simulink model "Block Diagram"  (R2024b)
settings: Solver=VariableStepAuto  StartTime=0.0  StopTime=10.0  RelTol=1e-3
libraries: simulink_extras x43, eeGeneralControl x4
(part 1 of 3)
settings Model: Creator=uig55046  LastModifiedBy=deepo
settings RTWCC: GPUComputeCapability=3.5

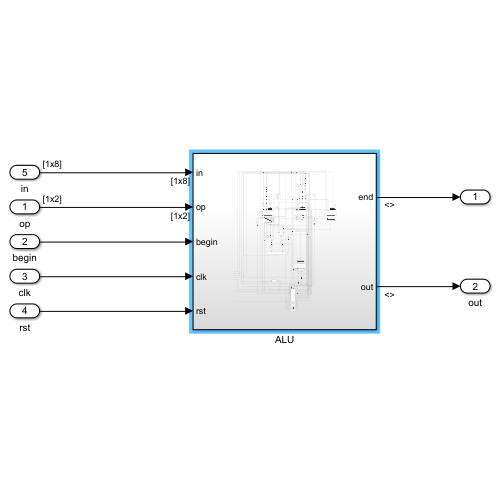
[thumbnail: Simulink's stored preview of the top-level diagram]
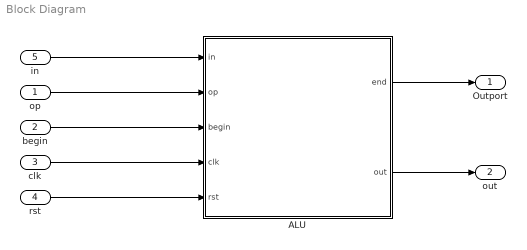
== system Block Diagram ==
  op : Inport  OutDataTypeStr=boolean  PortDimensions=[1 2]
  begin : Inport  Port=2  OutDataTypeStr=boolean  PortDimensions=[1]
      settings: VarSizeSig=Yes
  clk : Inport  Port=3  OutDataTypeStr=boolean  PortDimensions=1
  rst : Inport  Port=4
  in : Inport  Port=5  PortDimensions=[1 8]
  ALU : Subsystem
  Outport : Outport
  out : Outport  Port=2
  wires:
  op/1 -> ALU/2(op)
  begin/1 -> ALU/3(begin)
  clk/1 -> ALU/4(clk)
  ALU/1(end) -> Outport/1
  rst/1 -> ALU/5(rst)
  in/1 -> ALU/1(in)
  ALU/2(out) -> out/1

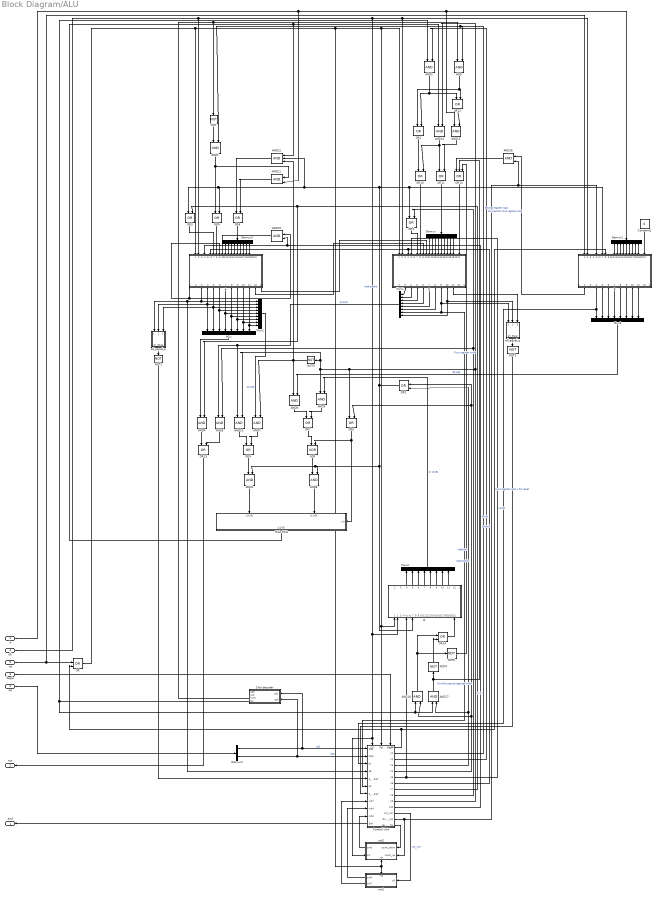
== system Block Diagram/ALU ==
  in : Inport  PortDimensions=[1 8]
  op : Inport  Port=2  PortDimensions=[1 2]
  begin : Inport  Port=3  PortDimensions=1  LockScale=on
  clk : Inport  Port=4
  rst : Inport  Port=5
  2-bit decoder : Subsystem
  9-bit RCA : Subsystem
      settings: PortSchema="{\"entries\":[{\"content\":{\"sides\":[{\"content\":{},\"type\":\"ConnectorPlacement.EquallySpacedRectSide\",\"uuid\":\"6c9f8647-f18e-41a6-b519-611a27a8b60b\"},{\"content\":{\"connectorIds\":[\"In3\"],\"side\":\"RIGHT\"},\"type\":\"ConnectorPlacement.EquallySpacedRectSide\",\"uuid\":\"5d0a121d-af89-432b-81b2-f63119ab70cd\"},{\"content\":{\"connectorIds\":[\"In1\",\"In2\"],\"side\":\"TOP\"},\"type\":\"ConnectorPlacement.EquallySpacedRectSide\",\"uuid\":\"30470a61-82f7-4402-b2c8-a4dff881e312\"},{\"content\":{\"connectorIds\":[\"Out1\"],\"side\":\"BOTTOM\"},\"type\":\"ConnectorPlacement.EquallySpacedRectSide\",\"uuid\":\"67fc6746-f29f-404d-858f-01e89e3881f2\"}]},\"type\":\"ConnectorPlacement.EquallySpacedConnector\",\"uuid\":\"99fec958-07ee-438f-8086-405a45e22bbf\"}],\"packageUris\":[\"http://schema.mathworks.com/mf0/Connector/R2020b\"],\"version\":\"1.0\"}"
  A : Subsystem
  AND{,1..11,13..18} (18 alike) : Logic  IconShape=distinctive  AllPortsSameDT=off  OutDataTypeStr=boolean
  AND12 : Logic  Inputs=3  IconShape=distinctive  AllPortsSameDT=off  OutDataTypeStr=boolean
  B : Subsystem
  Constant1 : Constant  Value=0
  Control Unit : Subsystem
      settings: PortSchema="{\"entries\":[{\"content\":{\"sides\":[{\"content\":{\"connectorIds\":[\"In1\",\"In2\",\"In3\",\"In4\",\"In5\",\"In6\",\"In7\",\"In8\",\"In9\",\"In10\",\"Out15\"]},\"type\":\"ConnectorPlacement.EquallySpacedRectSide\",\"uuid\":\"1c4597d9-3b0f-4cfb-b2e6-8dfea8a166b7\"},{\"content\":{\"connectorIds\":[\"Out1\",\"Out2\",\"Out3\",\"Out4\",\"Out5\",\"Out6\",\"Out7\",\"Out8\",\"Out9\",\"Out10\",\"Out11\",\"Out12\",\"Out13\",\"Out14\"],\"side\":\"RIGHT\"},\"type\":\"ConnectorPlacement.EquallySpacedRectSide\",\"uuid\":\"6c7a082a-77db-411d-a2a0-d4fa93b8c545\"},{\"content\":{\"connectorIds\":[\"In11\",\"In12\",\"In13\"],\"side\":\"TOP\"},\"type\":\"ConnectorPlacement.EquallySpacedRectSide\",\"uuid\":\"179b5546-1257-486e-9d19-cc9d48c86bde\"},{\"content\":{\"side\":\"BOTTOM\"},\"type\":\"ConnectorPlacement.EquallySpacedRectSide\",\"uuid\":\"abb4b6d3-db7d-4bb0-b032-1cb455e16e11\"}]},\"type\":\"ConnectorPlacement.EquallySpacedConnector\",\"uuid\":\"20d252ad-f679-4ef0-8503-9da12a7cac0d\"}],\"packageUris\":[\"http://schema.mathworks.com/mf0/Connector/R2020b\"],\"version\":\"1.0\"}"
  Demux : Demux  Outputs=9
  Demux1 : Demux  Outputs=9
  Demux2 : Demux  Outputs=2
  Demux3 : Demux  Outputs=9
  Mux{,1,3..4} (4 alike) : Mux  Inputs=8
  Mux2 : Mux  Inputs=9
  NOT{,1..5} (6 alike) : Logic  Operator=NOT  IconShape=distinctive  AllPortsSameDT=off  OutDataTypeStr=boolean
  OR{,1..12,14..15} (15 alike) : Logic  Operator=OR  IconShape=distinctive  AllPortsSameDT=off  OutDataTypeStr=boolean
  OR13 : Logic  Operator=OR  Inputs=3  IconShape=distinctive  AllPortsSameDT=off  OutDataTypeStr=boolean
  Q : Subsystem
  Q' : Subsystem
  XOR : Logic  Operator=XOR  IconShape=distinctive  AllPortsSameDT=off  OutDataTypeStr=boolean
  all_equal_a : Subsystem
  all_equal_q : Subsystem
  cnt1 : Subsystem
      settings: PortSchema="{\"entries\":[{\"content\":{\"sides\":[{\"content\":{\"connectorIds\":[\"In1\"]},\"type\":\"ConnectorPlacement.EquallySpacedRectSide\",\"uuid\":\"62ee226d-5239-4f1f-b580-7fc7b94eb7c9\"},{\"content\":{\"connectorIds\":[\"Out1\",\"Out2\"],\"side\":\"RIGHT\"},\"type\":\"ConnectorPlacement.EquallySpacedRectSide\",\"uuid\":\"b278d655-8a22-40b0-a666-39d0decd9fa0\"},{\"content\":{\"connectorIds\":[\"In2\"],\"side\":\"TOP\"},\"type\":\"ConnectorPlacement.EquallySpacedRectSide\",\"uuid\":\"accba41f-7684-4443-8feb-4325ee4f426e\"},{\"content\":{\"side\":\"BOTTOM\"},\"type\":\"ConnectorPlacement.EquallySpacedRectSide\",\"uuid\":\"009e46d0-0f6e-4762-8754-fc7f461e20dd\"}]},\"type\":\"ConnectorPlacement.EquallySpacedConnector\",\"uuid\":\"e4770ad1-5c71-4178-b13f-6abe5ba71a37\"}],\"packageUris\":[\"http://schema.mathworks.com/mf0/Connector/R2020b\"],\"version\":\"1.0\"}"
  cnt2 : Subsystem
      settings: PortSchema="{\"entries\":[{\"content\":{\"sides\":[{\"content\":{\"connectorIds\":[\"In1\",\"In2\"]},\"type\":\"ConnectorPlacement.EquallySpacedRectSide\",\"uuid\":\"f18e902a-c08d-4bfa-9b0d-72e50b289cdc\"},{\"content\":{\"connectorIds\":[\"Out1\",\"In4\"],\"side\":\"RIGHT\"},\"type\":\"ConnectorPlacement.EquallySpacedRectSide\",\"uuid\":\"816a8c59-597b-48e9-9305-be4463d611e7\"},{\"content\":{\"side\":\"TOP\"},\"type\":\"ConnectorPlacement.EquallySpacedRectSide\",\"uuid\":\"816e4885-608e-4562-a478-c3bb7c7eac08\"},{\"content\":{\"connectorIds\":[\"In3\"],\"side\":\"BOTTOM\"},\"type\":\"ConnectorPlacement.EquallySpacedRectSide\",\"uuid\":\"29cbdcff-a853-4ba2-969a-a459b73eb44c\"}]},\"type\":\"ConnectorPlacement.EquallySpacedConnector\",\"uuid\":\"8e8aef6c-f08c-4ce4-aec3-cbd2da88a560\"}],\"packageUris\":[\"http://schema.mathworks.com/mf0/Connector/R2020b\"],\"version\":\"1.0\"}"
  end : Outport
  out : Outport  Port=2
  wires:
  Demux/1 -> Q/11(b8)
  Demux/2 -> Q/12(b7)
  Demux/3 -> Q/13(b6)
  Demux/4 -> Q/14(b5)
  Demux/5 -> Q/15(b4)
  Demux/6 -> Q/16(b3)
  Demux/7 -> Q/17(b2)
  Demux/8 -> Q/18(b1)
  Demux/9 -> Q/19(b0)
  Demux1/1 -> B/11(b8)
  Demux1/2 -> B/12(b7)
  Demux1/3 -> B/13(b6)
  Demux1/4 -> B/14(b5)
  Demux1/5 -> B/15(b4)
  Demux1/6 -> B/16(b3)
  Demux1/7 -> B/17(b2)
  Demux1/8 -> B/18(b1)
  Demux1/9 -> B/19(b0)
  Control Unit/12(cnt_incr) -> cnt1/1(clk)  "cnt_incr"
  Control Unit/13(div_hold_init) -> AND16/2, B/5(ls), cnt2/2(count_up)
  Control Unit/14(div_hold_fin) -> cnt2/1(count_down)
  cnt1/1(cnt4) -> Control Unit/9(cnt4)
  cnt1/2(cnt7) -> Control Unit/8(cnt7)
  cnt2/1(cnt0) -> Control Unit/10(cnt0)
  clk/1 -> A/2(clk), Control Unit/11(Clk), cnt2/4(clk), Q'/2(clk), Q/2(clk), B/2(clk)
  begin/1 -> Control Unit/13(Begin)
  Control Unit/15(End) -> end/1
  op/1 -> Demux2/1
  Demux2/1 -> Control Unit/1(Op1), 2-bit decoder/1(op1)  "op1"
  Demux2/2 -> Control Unit/2(Op0), 2-bit decoder/2(op0)  "op0"
  Control Unit/9(c8) -> AND5/2, OR4/2  "Div/Mult second register write"
  Control Unit/8(c7) -> AND4/2, OR3/2  "First register write"
  Control Unit/6(c5) -> Q'/5(ls), Q/5(ls)  "Lshift"
  Control Unit/7(c6) -> Q/4(drs), A/6(rs)  "Rshfit"
  Control Unit/5(c4) -> AND18/2, OR6/2, OR2/1  "Subtraction"
  Control Unit/4(c3) -> OR2/2, AND17/2  "Addition"
  Control Unit/3(c2) -> AND2/2  "Div specific third register load"
  Control Unit/2(c1) -> AND1/2, AND/2  "Second register load"
  rst/1 -> OR/1, B/1(rst)
  Control Unit/1(c0) -> B/8(load), OR/2  "First register load + full reset"
  OR/1 -> A/1(rst), cnt1/2(rst), cnt2/3(rst), Control Unit/12(Rst), Q'/1(rst), Q/1(rst)
  2-bit decoder/3(mult) -> AND/1, NOT/1
  AND/1 -> OR1/1, OR12/2
  NOT/1 -> AND1/1
  OR1/1 -> OR10/1
  AND2/1 -> OR1/2, OR12/1
  2-bit decoder/4(div) -> AND17/1, AND18/1, AND2/1
  A/11(oub0) -> Mux/8, Mux2/9
  A/10(outb1) -> Mux/7, Mux2/8
  A/9(outb2) -> Mux/6, Mux2/7
  A/8(outb3) -> Mux/5, Mux2/6
  A/7(outb4) -> Mux/4, Mux2/5
  A/6(outb5) -> Mux/3, Mux2/4
  A/5(outb6) -> all_equal_a/3(in2), Mux/2, Mux2/3
  A/4(outb7) -> all_equal_a/2(in1), Mux/1, Mux2/2
  Q/3(outb8) -> Mux1/1
  Q/4(outb7) -> Mux1/2
  Q/5(outb6) -> Mux1/3
  Q/6(outb5) -> Mux1/4
  Q/7(outb4) -> Mux1/5
  Q/8(outb3) -> Mux1/6
  Q/10(outb1) -> all_equal_q/2(in1), Mux1/8
  A/3(outb8) -> all_equal_a/1(in0), Control Unit/4(a8), Mux2/1
  B/4(outb7) -> Mux3/1, Control Unit/3(b7)
  Q/9(outb2) -> Control Unit/6(q2), Mux1/7, all_equal_q/1(in0)
  all_equal_a/1(all_equal) -> NOT1/1
  NOT1/1 -> Control Unit/5(a_not_all_equal)
  all_equal_q/1(all_equal) -> NOT2/1
  Q/11(oub0) -> all_equal_q/3(in2)
  NOT2/1 -> Control Unit/7(q_not_all_equal)
  B/5(outb6) -> Mux3/2
  B/6(outb5) -> Mux3/3
  B/7(outb4) -> Mux3/4
  B/8(outb3) -> Mux3/5
  B/9(outb2) -> Mux3/6
  B/10(outb1) -> Mux3/7
  B/11(oub0) -> Mux3/8
  Mux3/1 -> AND8/2  "B[1x8]"
  Q'/4(outb7) -> Mux4/1
  Q'/5(outb6) -> Mux4/2
  Q'/6(outb5) -> Mux4/3
  Q'/7(outb4) -> Mux4/4
  Q'/8(outb3) -> Mux4/5
  Q'/9(outb2) -> Mux4/6
  Q'/10(outb1) -> Mux4/7
  Q'/11(oub0) -> Mux4/8
  Mux4/1 -> AND9/2  "Q`[1x8]"
  Mux/1 -> AND4/1
  AND4/1 -> OR15/1
  Mux1/1 -> AND10/1, AND5/1  "Q[1x8]"
  AND5/1 -> OR15/2
  OR3/1 -> A/7(write)
  Control Unit/10(c9) -> OR6/1, AND9/1, AND10/2, NOT3/1, AND14/2  "Q-Q`"
  OR6/1 -> XOR/2, 9-bit RCA/3(cin)
  OR2/1 -> OR9/2, OR3/1, AND12/2, OR4/1, B/7(write), AND3/2, AND6/2, Q'/7(write)  "load enable"
  AND8/1 -> OR7/1
  AND9/1 -> OR7/2
  NOT3/1 -> AND12/3, AND8/1, AND7/2
  OR7/1 -> XOR/1
  XOR/1 -> AND6/1
  AND6/1 -> 9-bit RCA/2(x[1x9])
  AND3/1 -> 9-bit RCA/1(y[1x9])
  OR4/1 -> Q/7(write)
  Mux2/1 -> AND7/1  "A[1x9]"
  OR5/1 -> AND3/1
  AND7/1 -> OR5/2
  AND10/1 -> OR5/1
  9-bit RCA/1(z[1x9]) -> AND12/1, AND14/1
  Demux3/9 -> A/19(b0)
  Demux3/8 -> A/18(b1)
  Demux3/7 -> A/17(b2)
  Demux3/6 -> A/16(b3)
  Demux3/5 -> A/15(b4)
  Demux3/4 -> A/14(b5)
  Demux3/3 -> A/13(b6)
  Demux3/2 -> A/12(b7)
  Demux3/1 -> A/11(b8)
  OR8/1 -> Demux3/1
  AND11/1 -> OR8/2
  AND12/1 -> OR8/1
  AND1/1 -> AND11/1, OR9/1
  OR9/1 -> A/8(load)
  OR10/1 -> Q/8(load)
  OR11/1 -> Demux/1
  AND14/1 -> OR10/2, OR11/1
  AND13/1 -> OR11/2
  OR12/1 -> AND13/2
  Control Unit/11(c10) -> AND15/2, A/4(drs)  "DRshift"
  A/1(iregbl1) -> AND15/1, A/9(oregbl1)
  AND15/1 -> A/10(oregbl0)
  A/13(iregbr0) -> Q/10(oregbl0)
  A/12(iregbr1) -> Q/9(oregbl1)
  B/2(iregbl0) -> AND16/1
  AND16/1 -> OR13/1
  Constant1/1 -> B/21(oregbr0)
  AND17/1 -> OR13/2, NOT4/1
  NOT4/1 -> OR14/2
  AND18/1 -> OR14/1, NOT5/1
  NOT5/1 -> OR13/3
  OR13/1 -> Q/21(oregbr0)
  OR14/1 -> Q'/21(oregbr0)
  in/1 -> AND11/2, AND13/1, Demux1/1
  OR15/1 -> out/1

== system Block Diagram/ALU/2-bit decoder ==
  op1 : Inport
  op0 : Inport  Port=2
  AND : Logic  IconShape=distinctive  AllPortsSameDT=off  OutDataTypeStr=boolean
  AND1 : Logic  IconShape=distinctive  AllPortsSameDT=off  OutDataTypeStr=boolean
  AND2 : Logic  IconShape=distinctive  AllPortsSameDT=off  OutDataTypeStr=boolean
  NOR : Logic  Operator=NOR  IconShape=distinctive  AllPortsSameDT=off  OutDataTypeStr=boolean
  NOT : Logic  Operator=NOT  IconShape=distinctive  AllPortsSameDT=off  OutDataTypeStr=boolean
  NOT1 : Logic  Operator=NOT  IconShape=distinctive  AllPortsSameDT=off  OutDataTypeStr=boolean
  add : Outport
  sub : Outport  Port=2
  mult : Outport  Port=3
  div : Outport  Port=4
  wires:
  NOR/1 -> add/1
  op1/1 -> AND2/1, AND1/1, NOT/1, NOR/1
  op0/1 -> AND/2, NOR/2, AND2/2, NOT1/1
  AND/1 -> sub/1
  NOT/1 -> AND/1
  AND1/1 -> mult/1
  NOT1/1 -> AND1/2
  AND2/1 -> div/1

== system Block Diagram/ALU/9-bit RCA ==
  y[1x9] : Inport
  x[1x9] : Inport  Port=2
  cin : Inport  Port=3
  9bitRCA : Subsystem
      settings: PortSchema="{\"entries\":[{\"content\":{\"sides\":[{\"content\":{},\"type\":\"ConnectorPlacement.EquallySpacedRectSide\",\"uuid\":\"72f60fbd-8b24-4db8-895c-c095f51eae04\"},{\"content\":{\"connectorIds\":[\"In19\"],\"side\":\"RIGHT\"},\"type\":\"ConnectorPlacement.EquallySpacedRectSide\",\"uuid\":\"0785d060-7a17-4f0a-a082-03ce6c5de10c\"},{\"content\":{\"connectorIds\":[\"In1\",\"In2\",\"In3\",\"In4\",\"In5\",\"In6\",\"In7\",\"In8\",\"In9\",\"In10\",\"In11\",\"In12\",\"In13\",\"In14\",\"In15\",\"In16\",\"In17\",\"In18\"],\"side\":\"TOP\"},\"type\":\"ConnectorPlacement.EquallySpacedRectSide\",\"uuid\":\"ef3cf86d-29e3-4c4c-9b85-b19d10bf65b5\"},{\"content\":{\"connectorIds\":[\"Out1\",\"Out2\",\"Out3\",\"Out4\",\"Out5\",\"Out6\",\"Out7\",\"Out8\",\"Out9\"],\"side\":\"BOTTOM\"},\"type\":\"ConnectorPlacement.EquallySpacedRectSide\",\"uuid\":\"6de85980-2cbf-4dba-ae6b-8e77b9f31f9f\"}]},\"type\":\"ConnectorPlacement.EquallySpacedConnector\",\"uuid\":\"0356d92d-5e40-4d9e-9dc4-32aef06e4ed2\"}],\"packageUris\":[\"http://schema.mathworks.com/mf0/Connector/R2020b\"],\"version\":\"1.0\"}"
  Demux1 : Demux  Outputs=9
  Demux2 : Demux  Outputs=9
  Mux2 : Mux  Inputs=9
  z[1x9] : Outport
  wires:
  x[1x9]/1 -> Demux2/1
  y[1x9]/1 -> Demux1/1
  Demux1/1 -> 9bitRCA/10(x8)
  Demux1/2 -> 9bitRCA/11(x7)
  Demux1/3 -> 9bitRCA/12(x6)
  Demux1/5 -> 9bitRCA/14(x4)
  Demux1/4 -> 9bitRCA/13(x5)
  Demux1/6 -> 9bitRCA/15(x3)
  Demux1/7 -> 9bitRCA/16(x2)
  Demux1/8 -> 9bitRCA/17(x1)
  Demux1/9 -> 9bitRCA/18(x0)
  Demux2/1 -> 9bitRCA/1(y8)
  Demux2/2 -> 9bitRCA/2(y7)
  Demux2/3 -> 9bitRCA/3(y6)
  Demux2/4 -> 9bitRCA/4(y5)
  Demux2/5 -> 9bitRCA/5(y4)
  Demux2/6 -> 9bitRCA/6(y3)
  Demux2/7 -> 9bitRCA/7(y2)
  Demux2/8 -> 9bitRCA/8(y1)
  Demux2/9 -> 9bitRCA/9(y0)
  9bitRCA/5(z4) -> Mux2/5
  9bitRCA/4(z5) -> Mux2/4
  9bitRCA/3(z6) -> Mux2/3
  9bitRCA/2(z7) -> Mux2/2
  9bitRCA/1(z8) -> Mux2/1
  9bitRCA/6(z3) -> Mux2/6
  9bitRCA/7(z2) -> Mux2/7
  9bitRCA/8(z1) -> Mux2/8
  9bitRCA/9(z0) -> Mux2/9
  Mux2/1 -> z[1x9]/1  "[1x9]"
  cin/1 -> 9bitRCA/19(cin)

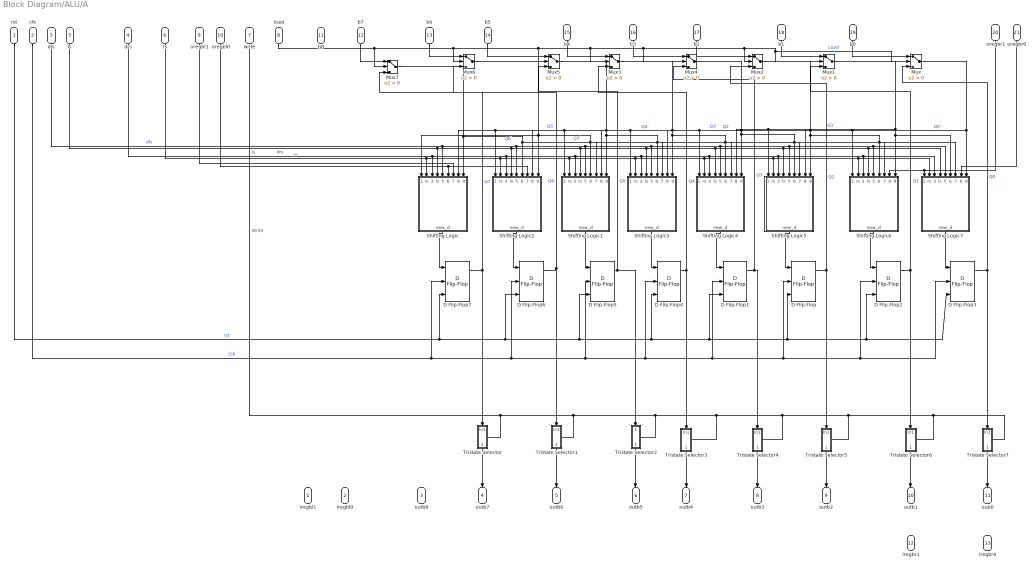
== system Block Diagram/ALU/A ==
  rst : Inport
  clk : Inport  Port=2
  dls : Inport  Port=3
  drs : Inport  Port=4
  ls : Inport  Port=5
  rs : Inport  Port=6
  write : Inport  Port=7
  load : Inport  Port=8
  oregbl1 : Inport  Port=9
  oregbl0 : Inport  Port=10
  b8 : Inport  Port=11
  b7 : Inport  Port=12
  b6 : Inport  Port=13
  b5 : Inport  Port=14
  b4 : Inport  Port=15
  b3 : Inport  Port=16
  b2 : Inport  Port=17
  b1 : Inport  Port=18
  b0 : Inport  Port=19
  oregbr1 : Inport  Port=20
  oregbr0 : Inport  Port=21
  D Flip-Flop{,1..7} (8 alike) : simulink_extras/Flip Flops/D Flip-Flop
  Mux{,1..7} (8 alike) : Switch  Criteria=u2 > Threshold  SaturateOnIntegerOverflow=off  InputSameDT=off
  Shifting Logic : Subsystem
  Shifting Logic1 : Subsystem
  Shifting Logic2 : Subsystem
  Shifting Logic3 : Subsystem
  Shifting Logic4 : Subsystem
  Shifting Logic5 : Subsystem
  Shifting Logic6 : Subsystem
  Shifting Logic7 : Subsystem
  Tristate Selector : Subsystem  TreatAsAtomicUnit=on
  Tristate Selector1 : Subsystem  TreatAsAtomicUnit=on
  Tristate Selector2 : Subsystem  TreatAsAtomicUnit=on
  Tristate Selector3 : Subsystem  TreatAsAtomicUnit=on
  Tristate Selector4 : Subsystem  TreatAsAtomicUnit=on
  Tristate Selector5 : Subsystem  TreatAsAtomicUnit=on
  Tristate Selector6 : Subsystem  TreatAsAtomicUnit=on
  Tristate Selector7 : Subsystem  TreatAsAtomicUnit=on
  iregbl1 : Outport
  iregbl0 : Outport  Port=2
  outb8 : Outport  Port=3
  outb7 : Outport  Port=4
  outb6 : Outport  Port=5
  outb5 : Outport  Port=6
  outb4 : Outport  Port=7
  outb3 : Outport  Port=8
  outb2 : Outport  Port=9
  outb1 : Outport  Port=10
  oub0 : Outport  Port=11
  iregbr1 : Outport  Port=12
  iregbr0 : Outport  Port=13
  wires:
  clk/1 -> D Flip-Flop5/2, D Flip-Flop4/2, D Flip-Flop1/2, D Flip-Flop/2, D Flip-Flop2/2, D Flip-Flop3/2, D Flip-Flop6/2, D Flip-Flop7/2  "Clk"
  b0/1 -> Mux/1
  b1/1 -> Mux1/1
  b2/1 -> Mux2/1
  b3/1 -> Mux4/1
  b4/1 -> Mux3/1
  b5/1 -> Mux5/1
  b6/1 -> Mux6/1
  b7/1 -> Mux7/1
  load/1 -> Mux5/2, Mux3/2, Mux4/2, Mux2/2, Mux1/2, Mux/2, Mux6/2, Mux7/2  "Load"
  D Flip-Flop7/1 -> Mux7/3, Tristate Selector/1(In1)  "Q7"
  D Flip-Flop6/1 -> Tristate Selector1/1(In1), Mux6/3  "Q6"
  D Flip-Flop5/1 -> Tristate Selector2/1(In1), Mux5/3  "Q5"
  D Flip-Flop4/1 -> Mux3/3, Tristate Selector3/1(In1)  "Q4"
  D Flip-Flop1/1 -> Tristate Selector4/1(In1), Mux4/3  "Q3"
  D Flip-Flop/1 -> Tristate Selector5/1(In1), Mux2/3  "Q2"
  D Flip-Flop2/1 -> Tristate Selector6/1(In1), Mux1/3  "Q1"
  D Flip-Flop3/1 -> Tristate Selector7/1(In1), Mux/3  "Q0"
  write/1 -> Tristate Selector/Action, Tristate Selector1/Action, Tristate Selector2/Action, Tristate Selector3/Action, Tristate Selector4/Action, Tristate Selector5/Action, Tristate Selector6/Action, Tristate Selector7/Action  "Write"
  Tristate Selector6/1(Out1) -> outb1/1
  Tristate Selector7/1(Out1) -> oub0/1
  Tristate Selector5/1(Out1) -> outb2/1
  Tristate Selector4/1(Out1) -> outb3/1
  Tristate Selector3/1(Out1) -> outb4/1
  Tristate Selector2/1(Out1) -> outb5/1
  Tristate Selector1/1(Out1) -> outb6/1
  Tristate Selector/1(Out1) -> outb7/1
  rst/1 -> D Flip-Flop7/3, D Flip-Flop4/3, D Flip-Flop/3, D Flip-Flop2/3, D Flip-Flop3/3, D Flip-Flop1/3, D Flip-Flop5/3, D Flip-Flop6/3  "rst"
  Mux6/1 -> Shifting Logic/1(lsb), Shifting Logic3/7(drsb), Shifting Logic1/6(rsb), Shifting Logic2/9(curr_b)  "Q6`"
  Mux2/1 -> Shifting Logic4/1(lsb), Shifting Logic3/8(dlsb), Shifting Logic7/7(drsb), Shifting Logic6/6(rsb), Shifting Logic5/9(curr_b)  "Q2`"
  Mux4/1 -> Shifting Logic1/8(dlsb), Shifting Logic3/1(lsb), Shifting Logic6/7(drsb), Shifting Logic5/6(rsb), Shifting Logic4/9(curr_b)  "Q3`"
  Mux3/1 -> Shifting Logic1/1(lsb), Shifting Logic2/8(dlsb), Shifting Logic5/7(drsb), Shifting Logic4/6(rsb), Shifting Logic3/9(curr_b)  "Q4`"
  Mux5/1 -> Shifting Logic/8(dlsb), Shifting Logic2/1(lsb), Shifting Logic4/7(drsb), Shifting Logic3/6(rsb), Shifting Logic1/9(curr_b)  "Q5`"
  Mux7/1 -> Shifting Logic1/7(drsb), Shifting Logic2/6(rsb), Shifting Logic/9(curr_b)  "Q7`"
  Shifting Logic/1(new_d) -> D Flip-Flop7/1
  Shifting Logic2/1(new_d) -> D Flip-Flop6/1
  Shifting Logic1/1(new_d) -> D Flip-Flop5/1
  Shifting Logic3/1(new_d) -> D Flip-Flop4/1
  Shifting Logic4/1(new_d) -> D Flip-Flop1/1
  Shifting Logic5/1(new_d) -> D Flip-Flop/1
  Shifting Logic6/1(new_d) -> D Flip-Flop2/1
  Shifting Logic7/1(new_d) -> D Flip-Flop3/1
  rs/1 -> Shifting Logic1/2(rs), Shifting Logic4/2(rs), Shifting Logic5/2(rs), Shifting Logic7/2(rs), Shifting Logic6/2(rs), Shifting Logic3/2(rs), Shifting Logic2/2(rs), Shifting Logic/2(rs)  "rs"
  drs/1 -> Shifting Logic/3(drs), Shifting Logic2/3(drs), Shifting Logic6/3(drs), Shifting Logic7/3(drs), Shifting Logic5/3(drs), Shifting Logic4/3(drs), Shifting Logic3/3(drs), Shifting Logic1/3(drs)  "drs"
  ls/1 -> Shifting Logic2/4(ls), Shifting Logic7/4(ls), Shifting Logic6/4(ls), Shifting Logic5/4(ls), Shifting Logic4/4(ls), Shifting Logic3/4(ls), Shifting Logic1/4(ls), Shifting Logic/4(ls)  "ls"
  dls/1 -> Shifting Logic1/5(dls), Shifting Logic3/5(dls), Shifting Logic4/5(dls), Shifting Logic5/5(dls), Shifting Logic6/5(dls), Shifting Logic7/5(dls), Shifting Logic2/5(dls), Shifting Logic/5(dls)  "dls"
  Mux1/1 -> Shifting Logic5/1(lsb), Shifting Logic4/8(dlsb), Shifting Logic7/6(rsb), Shifting Logic6/9(curr_b)  "Q1`"
  Mux/1 -> Shifting Logic6/1(lsb), Shifting Logic5/8(dlsb), Shifting Logic7/9(curr_b)  "Q0`"
  oregbr1/1 -> Shifting Logic6/8(dlsb), Shifting Logic7/1(lsb)
  oregbr0/1 -> Shifting Logic7/8(dlsb)
  oregbl0/1 -> Shifting Logic2/7(drsb), Shifting Logic/6(rsb)
  oregbl1/1 -> Shifting Logic/7(drsb)

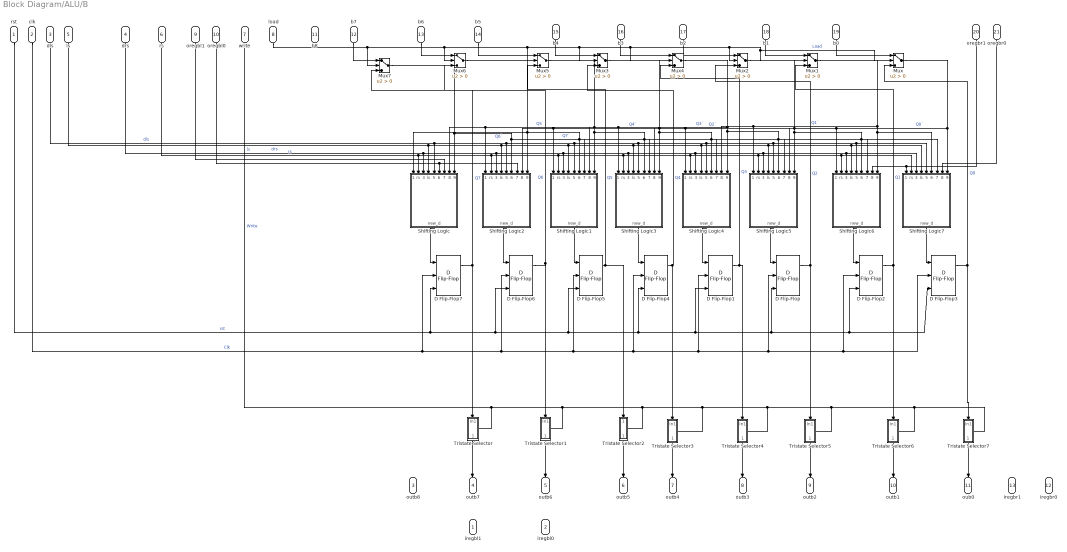
== system Block Diagram/ALU/B ==
  rst : Inport
  clk : Inport  Port=2
  dls : Inport  Port=3
  drs : Inport  Port=4
  ls : Inport  Port=5
  rs : Inport  Port=6
  write : Inport  Port=7
  load : Inport  Port=8
  oregbl1 : Inport  Port=9
  oregbl0 : Inport  Port=10
  b8 : Inport  Port=11
  b7 : Inport  Port=12
  b6 : Inport  Port=13
  b5 : Inport  Port=14
  b4 : Inport  Port=15
  b3 : Inport  Port=16
  b2 : Inport  Port=17
  b1 : Inport  Port=18
  b0 : Inport  Port=19
  oregbr1 : Inport  Port=20
  oregbr0 : Inport  Port=21
  D Flip-Flop{,1..7} (8 alike) : simulink_extras/Flip Flops/D Flip-Flop
  Mux{,1..7} (8 alike) : Switch  Criteria=u2 > Threshold  SaturateOnIntegerOverflow=off  InputSameDT=off
  Shifting Logic : Subsystem
  Shifting Logic1 : Subsystem
  Shifting Logic2 : Subsystem
  Shifting Logic3 : Subsystem
  Shifting Logic4 : Subsystem
  Shifting Logic5 : Subsystem
  Shifting Logic6 : Subsystem
  Shifting Logic7 : Subsystem
  Tristate Selector : Subsystem  TreatAsAtomicUnit=on
  Tristate Selector1 : Subsystem  TreatAsAtomicUnit=on
  Tristate Selector2 : Subsystem  TreatAsAtomicUnit=on
  Tristate Selector3 : Subsystem  TreatAsAtomicUnit=on
  Tristate Selector4 : Subsystem  TreatAsAtomicUnit=on
  Tristate Selector5 : Subsystem  TreatAsAtomicUnit=on
  Tristate Selector6 : Subsystem  TreatAsAtomicUnit=on
  Tristate Selector7 : Subsystem  TreatAsAtomicUnit=on
  iregbl1 : Outport
  iregbl0 : Outport  Port=2
  outb8 : Outport  Port=3
  outb7 : Outport  Port=4
  outb6 : Outport  Port=5
  outb5 : Outport  Port=6
  outb4 : Outport  Port=7
  outb3 : Outport  Port=8
  outb2 : Outport  Port=9
  outb1 : Outport  Port=10
  oub0 : Outport  Port=11
  iregbr0 : Outport  Port=12
  iregbr1 : Outport  Port=13
  wires:
  clk/1 -> D Flip-Flop5/2, D Flip-Flop4/2, D Flip-Flop1/2, D Flip-Flop/2, D Flip-Flop2/2, D Flip-Flop3/2, D Flip-Flop6/2, D Flip-Flop7/2  "Clk"
  b0/1 -> Mux/1
  b1/1 -> Mux1/1
  b2/1 -> Mux2/1
  b3/1 -> Mux4/1
  b4/1 -> Mux3/1
  b5/1 -> Mux5/1
  b6/1 -> Mux6/1
  b7/1 -> Mux7/1
  load/1 -> Mux5/2, Mux3/2, Mux4/2, Mux2/2, Mux1/2, Mux/2, Mux6/2, Mux7/2  "Load"
  D Flip-Flop7/1 -> Mux7/3, Tristate Selector/1(In1)  "Q7"
  D Flip-Flop6/1 -> Tristate Selector1/1(In1), Mux6/3  "Q6"
  D Flip-Flop5/1 -> Tristate Selector2/1(In1), Mux5/3  "Q5"
  D Flip-Flop4/1 -> Mux3/3, Tristate Selector3/1(In1)  "Q4"
  D Flip-Flop1/1 -> Tristate Selector4/1(In1), Mux4/3  "Q3"
  D Flip-Flop/1 -> Tristate Selector5/1(In1), Mux2/3  "Q2"
  D Flip-Flop2/1 -> Tristate Selector6/1(In1), Mux1/3  "Q1"
  D Flip-Flop3/1 -> Tristate Selector7/1(In1), Mux/3  "Q0"
  write/1 -> Tristate Selector/Action, Tristate Selector1/Action, Tristate Selector2/Action, Tristate Selector3/Action, Tristate Selector4/Action, Tristate Selector5/Action, Tristate Selector6/Action, Tristate Selector7/Action  "Write"
  Tristate Selector6/1(Out1) -> outb1/1
  Tristate Selector7/1(Out1) -> oub0/1
  Tristate Selector5/1(Out1) -> outb2/1
  Tristate Selector4/1(Out1) -> outb3/1
  Tristate Selector3/1(Out1) -> outb4/1
  Tristate Selector2/1(Out1) -> outb5/1
  Tristate Selector1/1(Out1) -> outb6/1
  Tristate Selector/1(Out1) -> outb7/1
  rst/1 -> D Flip-Flop7/3, D Flip-Flop4/3, D Flip-Flop/3, D Flip-Flop2/3, D Flip-Flop3/3, D Flip-Flop1/3, D Flip-Flop5/3, D Flip-Flop6/3  "rst"
  Mux6/1 -> Shifting Logic/1(lsb), Shifting Logic3/7(drsb), Shifting Logic1/6(rsb), Shifting Logic2/9(curr_b)  "Q6`"
  Mux2/1 -> Shifting Logic4/1(lsb), Shifting Logic3/8(dlsb), Shifting Logic7/7(drsb), Shifting Logic6/6(rsb), Shifting Logic5/9(curr_b)  "Q2`"
  Mux4/1 -> Shifting Logic1/8(dlsb), Shifting Logic3/1(lsb), Shifting Logic6/7(drsb), Shifting Logic5/6(rsb), Shifting Logic4/9(curr_b)  "Q3`"
  Mux3/1 -> Shifting Logic1/1(lsb), Shifting Logic2/8(dlsb), Shifting Logic5/7(drsb), Shifting Logic4/6(rsb), Shifting Logic3/9(curr_b)  "Q4`"
  Mux5/1 -> Shifting Logic/8(dlsb), Shifting Logic2/1(lsb), Shifting Logic4/7(drsb), Shifting Logic3/6(rsb), Shifting Logic1/9(curr_b)  "Q5`"
  Mux7/1 -> Shifting Logic1/7(drsb), Shifting Logic2/6(rsb), Shifting Logic/9(curr_b)  "Q7`"
  Shifting Logic/1(new_d) -> D Flip-Flop7/1
  Shifting Logic2/1(new_d) -> D Flip-Flop6/1
  Shifting Logic1/1(new_d) -> D Flip-Flop5/1
  Shifting Logic3/1(new_d) -> D Flip-Flop4/1
  Shifting Logic4/1(new_d) -> D Flip-Flop1/1
  Shifting Logic5/1(new_d) -> D Flip-Flop/1
  Shifting Logic6/1(new_d) -> D Flip-Flop2/1
  Shifting Logic7/1(new_d) -> D Flip-Flop3/1
  rs/1 -> Shifting Logic1/2(rs), Shifting Logic4/2(rs), Shifting Logic5/2(rs), Shifting Logic7/2(rs), Shifting Logic6/2(rs), Shifting Logic3/2(rs), Shifting Logic2/2(rs), Shifting Logic/2(rs)  "rs"
  drs/1 -> Shifting Logic/3(drs), Shifting Logic2/3(drs), Shifting Logic6/3(drs), Shifting Logic7/3(drs), Shifting Logic5/3(drs), Shifting Logic4/3(drs), Shifting Logic3/3(drs), Shifting Logic1/3(drs)  "drs"
  ls/1 -> Shifting Logic2/4(ls), Shifting Logic7/4(ls), Shifting Logic6/4(ls), Shifting Logic5/4(ls), Shifting Logic4/4(ls), Shifting Logic3/4(ls), Shifting Logic1/4(ls), Shifting Logic/4(ls)  "ls"
  dls/1 -> Shifting Logic1/5(dls), Shifting Logic3/5(dls), Shifting Logic4/5(dls), Shifting Logic5/5(dls), Shifting Logic6/5(dls), Shifting Logic7/5(dls), Shifting Logic2/5(dls), Shifting Logic/5(dls)  "dls"
  Mux1/1 -> Shifting Logic5/1(lsb), Shifting Logic4/8(dlsb), Shifting Logic7/6(rsb), Shifting Logic6/9(curr_b)  "Q1`"
  Mux/1 -> Shifting Logic6/1(lsb), Shifting Logic5/8(dlsb), Shifting Logic7/9(curr_b)  "Q0`"
  oregbr1/1 -> Shifting Logic6/8(dlsb), Shifting Logic7/1(lsb)
  oregbr0/1 -> Shifting Logic7/8(dlsb)
  oregbl0/1 -> Shifting Logic2/7(drsb), Shifting Logic/6(rsb)
  oregbl1/1 -> Shifting Logic/7(drsb)

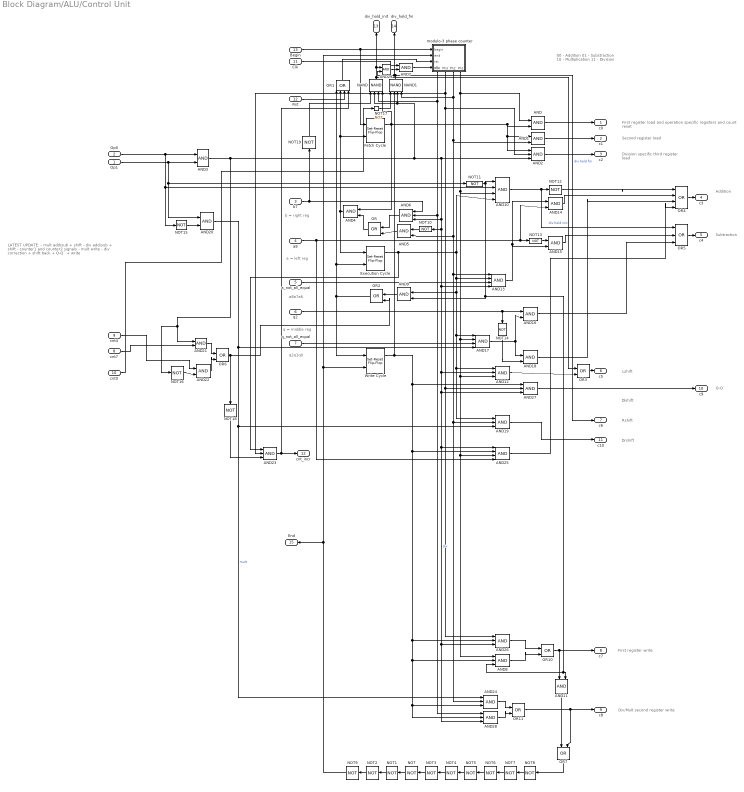
== system Block Diagram/ALU/Control Unit ==
  note: Q-Q`
  note: q2q1q0
  note: a8a7a6
  note: q = middle reg
  note: a = left reg
  note: b = right reg
  note: 00 - Addition
      | 01 - Substraction
      | 10 - Multiplication
      | 11 - Division
  note: Dlshift
  note: Subtraction
  note: Drshift
  note: Lshift
  note: Rshift
  note: Addition
  note: Division specific third register load
  note: Second register load
  note: First register load and operation specific registers and count reset
  note: First register write
  note: Div/Mult second register write
  note: LATEST UPDATE:
      | - mult add/sub + shift
      | - div add/sub + shift
      | - counter1 and counter2 signals
      | - mult write
      | - div correction + shift back + Q-Q` + write
  Op1 : Inport
  Op0 : Inport  Port=2
  b7 : Inport  Port=3
  a8 : Inport  Port=4
  a_not_all_equal : Inport  Port=5
  q2 : Inport  Port=6
  q_not_all_equal : Inport  Port=7
  cnt7 : Inport  Port=8
  cnt4 : Inport  Port=9
  cnt0 : Inport  Port=10
  Clk : Inport  Port=11
  Rst : Inport  Port=12
  Begin : Inport  Port=13
  AND{,1,3..5,7,9,11,14..16,18,20..22,29} (16 alike) : Logic  IconShape=distinctive  AllPortsSameDT=off  OutDataTypeStr=boolean
  AND{10,13,17,25} (4 alike) : Logic  Inputs=4  IconShape=distinctive  AllPortsSameDT=off  OutDataTypeStr=boolean
  AND{2,6,8,12,19,23..24,26..28} (10 alike) : Logic  Inputs=3  IconShape=distinctive  AllPortsSameDT=off  OutDataTypeStr=boolean
  Execution Cycle : eeGeneralControl/Set-Reset Flip-Flop  LabelModeActiveChoice=Discrete  UndefState=Set  Q0=0  Ts=-1
      settings: LibrarySourceBlock=ee_sl_lib/General Control/Set-Reset Flip-Flop
  Fetch Cycle : eeGeneralControl/Set-Reset Flip-Flop  LabelModeActiveChoice=Discrete  UndefState=Set  Q0=0  Ts=-1
      settings: LibrarySourceBlock=ee_sl_lib/General Control/Set-Reset Flip-Flop
  NAND : Logic  Operator=NAND  Inputs=4  IconShape=distinctive  AllPortsSameDT=off  OutDataTypeStr=boolean
  NAND1 : Logic  Operator=NAND  Inputs=4  IconShape=distinctive  AllPortsSameDT=off  OutDataTypeStr=boolean
  NOT{,1..19} (20 alike) : Logic  Operator=NOT  IconShape=distinctive  AllPortsSameDT=off  OutDataTypeStr=boolean
  OR{,2..3,6..7,10..11} (7 alike) : Logic  Operator=OR  IconShape=distinctive  AllPortsSameDT=off  OutDataTypeStr=boolean
  OR1 : Logic  Operator=OR  Inputs=4  IconShape=distinctive  AllPortsSameDT=off  OutDataTypeStr=boolean
  OR4 : Logic  Operator=OR  Inputs=4  IconShape=distinctive  AllPortsSameDT=off  OutDataTypeStr=boolean
  OR5 : Logic  Operator=OR  Inputs=3  IconShape=distinctive  AllPortsSameDT=off  OutDataTypeStr=boolean
  Write Cycle : eeGeneralControl/Set-Reset Flip-Flop  LabelModeActiveChoice=Discrete  UndefState=Set  Q0=0  Ts=-1
      settings: LibrarySourceBlock=ee_sl_lib/General Control/Set-Reset Flip-Flop
  modulo-3 phase counter : Subsystem
      settings: PortSchema="{\"entries\":[{\"content\":{\"sides\":[{\"content\":{\"connectorIds\":[\"In1\",\"In2\",\"In3\",\"In4\"]},\"type\":\"ConnectorPlacement.EquallySpacedRectSide\",\"uuid\":\"a8b117dd-2946-49ef-bbed-ae3cc108d11e\"},{\"content\":{\"side\":\"RIGHT\"},\"type\":\"ConnectorPlacement.EquallySpacedRectSide\",\"uuid\":\"bacd4760-4572-4b2b-9826-237cfdf894e3\"},{\"content\":{\"side\":\"TOP\"},\"type\":\"ConnectorPlacement.EquallySpacedRectSide\",\"uuid\":\"eaf2d0ed-48ce-4eb0-81f0-946105eac7cf\"},{\"content\":{\"connectorIds\":[\"Out1\",\"Out2\",\"Out3\",\"Out4\"],\"side\":\"BOTTOM\"},\"type\":\"ConnectorPlacement.EquallySpacedRectSide\",\"uuid\":\"a9f9fcfc-78b5-4f50-a085-01a07af4e39a\"}]},\"type\":\"ConnectorPlacement.EquallySpacedConnector\",\"uuid\":\"ddf40ff0-bdf4-443c-9a95-5c8276050d8f\"}],\"packageUris\":[\"http://schema.mathworks.com/mf0/Connector/R2020b\"],\"version\":\"1.0\"}"
  c0 : Outport
  c1 : Outport  Port=2
  c2 : Outport  Port=3
  c3 : Outport  Port=4
  c4 : Outport  Port=5
  c5 : Outport  Port=6
  c6 : Outport  Port=7
  c7 : Outport  Port=8
  c8 : Outport  Port=9
  c9 : Outport  Port=10
  c10 : Outport  Port=11
  cnt_incr : Outport  Port=12
  div_hold_init : Outport  Port=13
  div_hold_fin : Outport  Port=14
  End : Outport  Port=15
  wires:
  NOT9/1 -> modulo-3 phase counter/2(end), Write Cycle/2, End/1
  Begin/1 -> Fetch Cycle/1, modulo-3 phase counter/1(begin)
  Fetch Cycle/1 -> AND4/1, NAND/4, AND2/1, AND1/1, AND/2
  AND/1 -> c0/1
  modulo-3 phase counter/3(Ph2) -> NAND1/4, AND24/2, AND19/2, AND13/1, AND5/2, AND1/2
  AND1/1 -> c1/1
  modulo-3 phase counter/2(Ph3) -> AND27/2, AND26/1, AND2/2, AND23/2
  AND3/1 -> AND2/3, AND13/4, AND27/3, AND25/1, AND26/3, AND28/3, AND12/2, NOT10/1, AND6/3, NAND1/3, NAND/2, NOT16/1, AND21/1  "div"
  AND2/1 -> c2/1
  NOT8/1 -> NOT7/1
  NOT7/1 -> NOT6/1
  NOT6/1 -> NOT5/1
  NOT5/1 -> NOT4/1
  NOT3/1 -> NOT/1
  NOT/1 -> NOT1/1
  NOT1/1 -> NOT2/1
  NOT2/1 -> NOT9/1
  NOT4/1 -> NOT3/1
  AND4/1 -> Execution Cycle/1, Fetch Cycle/2, OR1/2
  AND5/1 -> OR/2
  AND6/1 -> OR/1
  OR/1 -> AND4/2
  NOT10/1 -> AND5/1
  modulo-3 phase counter/1(Ph4) -> AND28/1, AND6/2, NAND/3
  b7/1 -> AND6/1, NOT19/1
  Clk/1 -> AND7/1
  AND7/1 -> modulo-3 phase counter/4(clk)
  NAND/1 -> OR3/1, AND29/1, div_hold_init/1  "div hold init"
  Rst/1 -> OR1/3
  OR1/1 -> modulo-3 phase counter/3(rst)
  Op0/1 -> AND3/1, NOT15/1, AND10/2
  Op1/1 -> AND3/2, AND20/1, NOT11/1
  AND10/1 -> OR5/1, NOT12/1
  NOT12/1 -> OR4/1
  Execution Cycle/1 -> AND23/1, AND19/1, AND12/1, AND17/1, AND9/1, AND13/2, AND10/4
  AND9/1 -> OR2/1
  OR2/1 -> OR1/1, Execution Cycle/2, Write Cycle/1
  AND8/1 -> OR10/2
  Write Cycle/1 -> NAND1/2, AND28/2, AND24/3, AND8/2, AND26/2, AND25/2, AND27/1
  NOT11/1 -> AND9/2, AND8/3, AND11/2, AND10/1
  modulo-3 phase counter/4(Ph1) -> AND8/1, AND25/3, AND12/3, AND17/2, AND10/3, AND/1
  AND12/1 -> OR3/2
  OR3/1 -> c5/1
  a_not_all_equal/1 -> AND13/3
  a8/1 -> AND25/4, NOT13/1, AND14/2
  AND13/1 -> AND15/2, AND14/1
  NOT13/1 -> AND15/1
  OR4/1 -> c3/1
  AND14/1 -> OR4/2
  OR5/1 -> c4/1
  AND15/1 -> OR5/2
  q_not_all_equal/1 -> AND17/3
  AND17/1 -> AND18/1, AND16/2
  q2/1 -> AND16/1, NOT14/1
  AND16/1 -> OR5/3
  NOT14/1 -> AND18/2
  AND18/1 -> OR4/3
  NOT15/1 -> AND20/2
  AND20/1 -> AND19/3, AND24/1, AND17/4  "mult"
  AND19/1 -> c10/1
  cnt7/1 -> AND21/2
  cnt4/1 -> AND22/1
  NOT16/1 -> AND22/2
  AND21/1 -> OR6/1
  AND22/1 -> OR6/2
  OR6/1 -> OR2/2, NOT18/1
  NOT18/1 -> AND23/3
  AND23/1 -> cnt_incr/1, OR1/4
  OR10/1 -> c7/1, AND11/1
  OR7/1 -> NOT8/1
  AND25/1 -> OR4/4
  AND29/1 -> AND7/2
  NAND1/1 -> c6/1, div_hold_fin/1, AND29/2  "div hold fin"
  NOT17/1 -> NAND1/1
  cnt0/1 -> NOT17/1
  AND26/1 -> OR10/1
  AND27/1 -> c9/1
  AND24/1 -> OR11/1
  OR11/1 -> OR7/2, c8/1
  AND28/1 -> OR11/2
  NOT19/1 -> NAND/1
  AND11/1 -> OR7/1

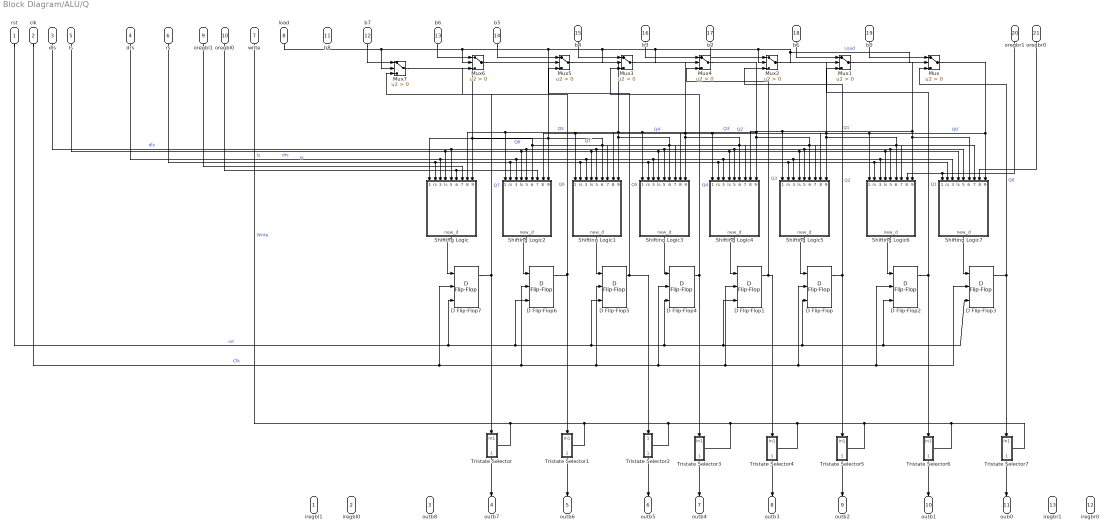
== system Block Diagram/ALU/Q ==
  rst : Inport
  clk : Inport  Port=2
  dls : Inport  Port=3
  drs : Inport  Port=4
  ls : Inport  Port=5
  rs : Inport  Port=6
  write : Inport  Port=7
  load : Inport  Port=8
  oregbl1 : Inport  Port=9
  oregbl0 : Inport  Port=10
  b8 : Inport  Port=11
  b7 : Inport  Port=12
  b6 : Inport  Port=13
  b5 : Inport  Port=14
  b4 : Inport  Port=15
  b3 : Inport  Port=16
  b2 : Inport  Port=17
  b1 : Inport  Port=18
  b0 : Inport  Port=19
  oregbr1 : Inport  Port=20
  oregbr0 : Inport  Port=21
  D Flip-Flop{,1..7} (8 alike) : simulink_extras/Flip Flops/D Flip-Flop
  Mux{,1..7} (8 alike) : Switch  Criteria=u2 > Threshold  SaturateOnIntegerOverflow=off  InputSameDT=off
  Shifting Logic : Subsystem
  Shifting Logic1 : Subsystem
  Shifting Logic2 : Subsystem
  Shifting Logic3 : Subsystem
  Shifting Logic4 : Subsystem
  Shifting Logic5 : Subsystem
  Shifting Logic6 : Subsystem
  Shifting Logic7 : Subsystem
  Tristate Selector : Subsystem  TreatAsAtomicUnit=on
  Tristate Selector1 : Subsystem  TreatAsAtomicUnit=on
  Tristate Selector2 : Subsystem  TreatAsAtomicUnit=on
  Tristate Selector3 : Subsystem  TreatAsAtomicUnit=on
  Tristate Selector4 : Subsystem  TreatAsAtomicUnit=on
  Tristate Selector5 : Subsystem  TreatAsAtomicUnit=on
  Tristate Selector6 : Subsystem  TreatAsAtomicUnit=on
  Tristate Selector7 : Subsystem  TreatAsAtomicUnit=on
  iregbl1 : Outport
  iregbl0 : Outport  Port=2
  outb8 : Outport  Port=3
  outb7 : Outport  Port=4
  outb6 : Outport  Port=5
  outb5 : Outport  Port=6
  outb4 : Outport  Port=7
  outb3 : Outport  Port=8
  outb2 : Outport  Port=9
  outb1 : Outport  Port=10
  oub0 : Outport  Port=11
  iregbr0 : Outport  Port=12
  iregbr1 : Outport  Port=13
  wires:
  clk/1 -> D Flip-Flop5/2, D Flip-Flop4/2, D Flip-Flop1/2, D Flip-Flop/2, D Flip-Flop2/2, D Flip-Flop3/2, D Flip-Flop6/2, D Flip-Flop7/2  "Clk"
  b0/1 -> Mux/1
  b1/1 -> Mux1/1
  b2/1 -> Mux2/1
  b3/1 -> Mux4/1
  b4/1 -> Mux3/1
  b5/1 -> Mux5/1
  b6/1 -> Mux6/1
  b7/1 -> Mux7/1
  load/1 -> Mux5/2, Mux3/2, Mux4/2, Mux2/2, Mux1/2, Mux/2, Mux6/2, Mux7/2  "Load"
  D Flip-Flop7/1 -> Mux7/3, Tristate Selector/1(In1)  "Q7"
  D Flip-Flop6/1 -> Tristate Selector1/1(In1), Mux6/3  "Q6"
  D Flip-Flop5/1 -> Tristate Selector2/1(In1), Mux5/3  "Q5"
  D Flip-Flop4/1 -> Mux3/3, Tristate Selector3/1(In1)  "Q4"
  D Flip-Flop1/1 -> Tristate Selector4/1(In1), Mux4/3  "Q3"
  D Flip-Flop/1 -> Tristate Selector5/1(In1), Mux2/3  "Q2"
  D Flip-Flop2/1 -> Tristate Selector6/1(In1), Mux1/3  "Q1"
  D Flip-Flop3/1 -> Tristate Selector7/1(In1), Mux/3  "Q0"
  write/1 -> Tristate Selector/Action, Tristate Selector1/Action, Tristate Selector2/Action, Tristate Selector3/Action, Tristate Selector4/Action, Tristate Selector5/Action, Tristate Selector6/Action, Tristate Selector7/Action  "Write"
  Tristate Selector6/1(Out1) -> outb1/1
  Tristate Selector7/1(Out1) -> oub0/1
  Tristate Selector5/1(Out1) -> outb2/1
  Tristate Selector4/1(Out1) -> outb3/1
  Tristate Selector3/1(Out1) -> outb4/1
  Tristate Selector2/1(Out1) -> outb5/1
  Tristate Selector1/1(Out1) -> outb6/1
  Tristate Selector/1(Out1) -> outb7/1
  rst/1 -> D Flip-Flop7/3, D Flip-Flop4/3, D Flip-Flop/3, D Flip-Flop2/3, D Flip-Flop3/3, D Flip-Flop1/3, D Flip-Flop5/3, D Flip-Flop6/3  "rst"
  Mux6/1 -> Shifting Logic/1(lsb), Shifting Logic3/7(drsb), Shifting Logic1/6(rsb), Shifting Logic2/9(curr_b)  "Q6`"
  Mux2/1 -> Shifting Logic4/1(lsb), Shifting Logic3/8(dlsb), Shifting Logic7/7(drsb), Shifting Logic6/6(rsb), Shifting Logic5/9(curr_b)  "Q2`"
  Mux4/1 -> Shifting Logic1/8(dlsb), Shifting Logic3/1(lsb), Shifting Logic6/7(drsb), Shifting Logic5/6(rsb), Shifting Logic4/9(curr_b)  "Q3`"
  Mux3/1 -> Shifting Logic1/1(lsb), Shifting Logic2/8(dlsb), Shifting Logic5/7(drsb), Shifting Logic4/6(rsb), Shifting Logic3/9(curr_b)  "Q4`"
  Mux5/1 -> Shifting Logic/8(dlsb), Shifting Logic2/1(lsb), Shifting Logic4/7(drsb), Shifting Logic3/6(rsb), Shifting Logic1/9(curr_b)  "Q5`"
  Mux7/1 -> Shifting Logic1/7(drsb), Shifting Logic2/6(rsb), Shifting Logic/9(curr_b)  "Q7`"
  Shifting Logic/1(new_d) -> D Flip-Flop7/1
  Shifting Logic2/1(new_d) -> D Flip-Flop6/1
  Shifting Logic1/1(new_d) -> D Flip-Flop5/1
  Shifting Logic3/1(new_d) -> D Flip-Flop4/1
  Shifting Logic4/1(new_d) -> D Flip-Flop1/1
  Shifting Logic5/1(new_d) -> D Flip-Flop/1
  Shifting Logic6/1(new_d) -> D Flip-Flop2/1
  Shifting Logic7/1(new_d) -> D Flip-Flop3/1
  rs/1 -> Shifting Logic1/2(rs), Shifting Logic4/2(rs), Shifting Logic5/2(rs), Shifting Logic7/2(rs), Shifting Logic6/2(rs), Shifting Logic3/2(rs), Shifting Logic2/2(rs), Shifting Logic/2(rs)  "rs"
  drs/1 -> Shifting Logic/3(drs), Shifting Logic2/3(drs), Shifting Logic6/3(drs), Shifting Logic7/3(drs), Shifting Logic5/3(drs), Shifting Logic4/3(drs), Shifting Logic3/3(drs), Shifting Logic1/3(drs)  "drs"
  ls/1 -> Shifting Logic2/4(ls), Shifting Logic7/4(ls), Shifting Logic6/4(ls), Shifting Logic5/4(ls), Shifting Logic4/4(ls), Shifting Logic3/4(ls), Shifting Logic1/4(ls), Shifting Logic/4(ls)  "ls"
  dls/1 -> Shifting Logic1/5(dls), Shifting Logic3/5(dls), Shifting Logic4/5(dls), Shifting Logic5/5(dls), Shifting Logic6/5(dls), Shifting Logic7/5(dls), Shifting Logic2/5(dls), Shifting Logic/5(dls)  "dls"
  Mux1/1 -> Shifting Logic5/1(lsb), Shifting Logic4/8(dlsb), Shifting Logic7/6(rsb), Shifting Logic6/9(curr_b)  "Q1`"
  Mux/1 -> Shifting Logic6/1(lsb), Shifting Logic5/8(dlsb), Shifting Logic7/9(curr_b)  "Q0`"
  oregbr1/1 -> Shifting Logic6/8(dlsb), Shifting Logic7/1(lsb)
  oregbr0/1 -> Shifting Logic7/8(dlsb)
  oregbl0/1 -> Shifting Logic2/7(drsb), Shifting Logic/6(rsb)
  oregbl1/1 -> Shifting Logic/7(drsb)

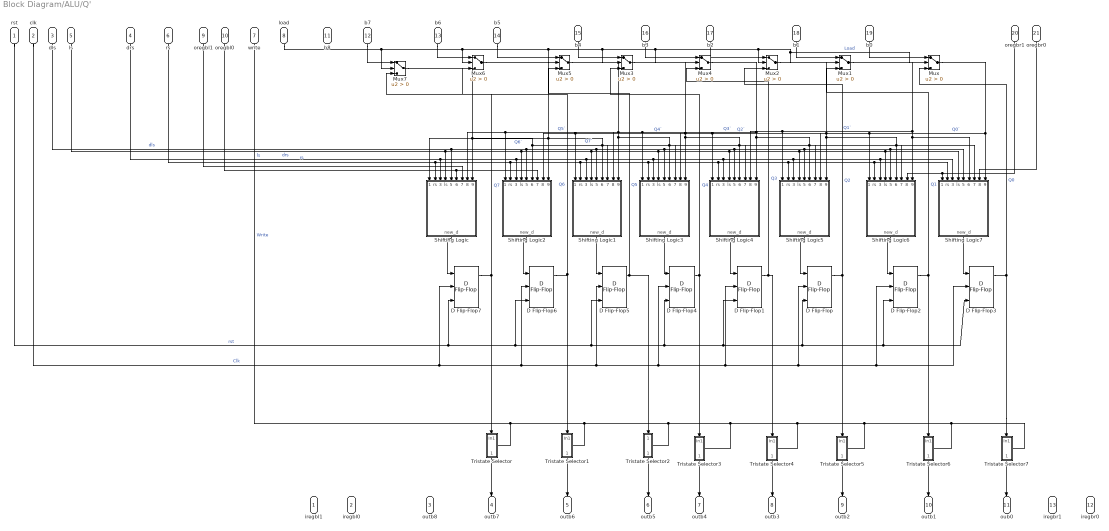
== system Block Diagram/ALU/Q' ==
  rst : Inport
  clk : Inport  Port=2
  dls : Inport  Port=3
  drs : Inport  Port=4
  ls : Inport  Port=5
  rs : Inport  Port=6
  write : Inport  Port=7
  load : Inport  Port=8
  oregbl1 : Inport  Port=9
  oregbl0 : Inport  Port=10
  b8 : Inport  Port=11
  b7 : Inport  Port=12
  b6 : Inport  Port=13
  b5 : Inport  Port=14
  b4 : Inport  Port=15
  b3 : Inport  Port=16
  b2 : Inport  Port=17
  b1 : Inport  Port=18
  b0 : Inport  Port=19
  oregbr1 : Inport  Port=20
  oregbr0 : Inport  Port=21
  D Flip-Flop{,1..7} (8 alike) : simulink_extras/Flip Flops/D Flip-Flop
  Mux{,1..7} (8 alike) : Switch  Criteria=u2 > Threshold  SaturateOnIntegerOverflow=off  InputSameDT=off
  Shifting Logic : Subsystem
  Shifting Logic1 : Subsystem
  Shifting Logic2 : Subsystem
  Shifting Logic3 : Subsystem
  Shifting Logic4 : Subsystem
  Shifting Logic5 : Subsystem
  Shifting Logic6 : Subsystem
  Shifting Logic7 : Subsystem
  Tristate Selector : Subsystem  TreatAsAtomicUnit=on
  Tristate Selector1 : Subsystem  TreatAsAtomicUnit=on
  Tristate Selector2 : Subsystem  TreatAsAtomicUnit=on
  Tristate Selector3 : Subsystem  TreatAsAtomicUnit=on
  Tristate Selector4 : Subsystem  TreatAsAtomicUnit=on
  Tristate Selector5 : Subsystem  TreatAsAtomicUnit=on
  Tristate Selector6 : Subsystem  TreatAsAtomicUnit=on
  Tristate Selector7 : Subsystem  TreatAsAtomicUnit=on
  iregbl1 : Outport
  iregbl0 : Outport  Port=2
  outb8 : Outport  Port=3
  outb7 : Outport  Port=4
  outb6 : Outport  Port=5
  outb5 : Outport  Port=6
  outb4 : Outport  Port=7
  outb3 : Outport  Port=8
  outb2 : Outport  Port=9
  outb1 : Outport  Port=10
  oub0 : Outport  Port=11
  iregbr0 : Outport  Port=12
  iregbr1 : Outport  Port=13
  wires:
  clk/1 -> D Flip-Flop5/2, D Flip-Flop4/2, D Flip-Flop1/2, D Flip-Flop/2, D Flip-Flop2/2, D Flip-Flop3/2, D Flip-Flop6/2, D Flip-Flop7/2  "Clk"
  b0/1 -> Mux/1
  b1/1 -> Mux1/1
  b2/1 -> Mux2/1
  b3/1 -> Mux4/1
  b4/1 -> Mux3/1
  b5/1 -> Mux5/1
  b6/1 -> Mux6/1
  b7/1 -> Mux7/1
  load/1 -> Mux5/2, Mux3/2, Mux4/2, Mux2/2, Mux1/2, Mux/2, Mux6/2, Mux7/2  "Load"
  D Flip-Flop7/1 -> Mux7/3, Tristate Selector/1(In1)  "Q7"
  D Flip-Flop6/1 -> Tristate Selector1/1(In1), Mux6/3  "Q6"
  D Flip-Flop5/1 -> Tristate Selector2/1(In1), Mux5/3  "Q5"
  D Flip-Flop4/1 -> Mux3/3, Tristate Selector3/1(In1)  "Q4"
  D Flip-Flop1/1 -> Tristate Selector4/1(In1), Mux4/3  "Q3"
  D Flip-Flop/1 -> Tristate Selector5/1(In1), Mux2/3  "Q2"
  D Flip-Flop2/1 -> Tristate Selector6/1(In1), Mux1/3  "Q1"
  D Flip-Flop3/1 -> Tristate Selector7/1(In1), Mux/3  "Q0"
  write/1 -> Tristate Selector/Action, Tristate Selector1/Action, Tristate Selector2/Action, Tristate Selector3/Action, Tristate Selector4/Action, Tristate Selector5/Action, Tristate Selector6/Action, Tristate Selector7/Action  "Write"
  Tristate Selector6/1(Out1) -> outb1/1
  Tristate Selector7/1(Out1) -> oub0/1
  Tristate Selector5/1(Out1) -> outb2/1
  Tristate Selector4/1(Out1) -> outb3/1
  Tristate Selector3/1(Out1) -> outb4/1
  Tristate Selector2/1(Out1) -> outb5/1
  Tristate Selector1/1(Out1) -> outb6/1
  Tristate Selector/1(Out1) -> outb7/1
  rst/1 -> D Flip-Flop7/3, D Flip-Flop4/3, D Flip-Flop/3, D Flip-Flop2/3, D Flip-Flop3/3, D Flip-Flop1/3, D Flip-Flop5/3, D Flip-Flop6/3  "rst"
  Mux6/1 -> Shifting Logic/1(lsb), Shifting Logic3/7(drsb), Shifting Logic1/6(rsb), Shifting Logic2/9(curr_b)  "Q6`"
  Mux2/1 -> Shifting Logic4/1(lsb), Shifting Logic3/8(dlsb), Shifting Logic7/7(drsb), Shifting Logic6/6(rsb), Shifting Logic5/9(curr_b)  "Q2`"
  Mux4/1 -> Shifting Logic1/8(dlsb), Shifting Logic3/1(lsb), Shifting Logic6/7(drsb), Shifting Logic5/6(rsb), Shifting Logic4/9(curr_b)  "Q3`"
  Mux3/1 -> Shifting Logic1/1(lsb), Shifting Logic2/8(dlsb), Shifting Logic5/7(drsb), Shifting Logic4/6(rsb), Shifting Logic3/9(curr_b)  "Q4`"
  Mux5/1 -> Shifting Logic/8(dlsb), Shifting Logic2/1(lsb), Shifting Logic4/7(drsb), Shifting Logic3/6(rsb), Shifting Logic1/9(curr_b)  "Q5`"
  Mux7/1 -> Shifting Logic1/7(drsb), Shifting Logic2/6(rsb), Shifting Logic/9(curr_b)  "Q7`"
  Shifting Logic/1(new_d) -> D Flip-Flop7/1
  Shifting Logic2/1(new_d) -> D Flip-Flop6/1
  Shifting Logic1/1(new_d) -> D Flip-Flop5/1
  Shifting Logic3/1(new_d) -> D Flip-Flop4/1
  Shifting Logic4/1(new_d) -> D Flip-Flop1/1
  Shifting Logic5/1(new_d) -> D Flip-Flop/1
  Shifting Logic6/1(new_d) -> D Flip-Flop2/1
  Shifting Logic7/1(new_d) -> D Flip-Flop3/1
  rs/1 -> Shifting Logic1/2(rs), Shifting Logic4/2(rs), Shifting Logic5/2(rs), Shifting Logic7/2(rs), Shifting Logic6/2(rs), Shifting Logic3/2(rs), Shifting Logic2/2(rs), Shifting Logic/2(rs)  "rs"
  drs/1 -> Shifting Logic/3(drs), Shifting Logic2/3(drs), Shifting Logic6/3(drs), Shifting Logic7/3(drs), Shifting Logic5/3(drs), Shifting Logic4/3(drs), Shifting Logic3/3(drs), Shifting Logic1/3(drs)  "drs"
  ls/1 -> Shifting Logic2/4(ls), Shifting Logic7/4(ls), Shifting Logic6/4(ls), Shifting Logic5/4(ls), Shifting Logic4/4(ls), Shifting Logic3/4(ls), Shifting Logic1/4(ls), Shifting Logic/4(ls)  "ls"
  dls/1 -> Shifting Logic1/5(dls), Shifting Logic3/5(dls), Shifting Logic4/5(dls), Shifting Logic5/5(dls), Shifting Logic6/5(dls), Shifting Logic7/5(dls), Shifting Logic2/5(dls), Shifting Logic/5(dls)  "dls"
  Mux1/1 -> Shifting Logic5/1(lsb), Shifting Logic4/8(dlsb), Shifting Logic7/6(rsb), Shifting Logic6/9(curr_b)  "Q1`"
  Mux/1 -> Shifting Logic6/1(lsb), Shifting Logic5/8(dlsb), Shifting Logic7/9(curr_b)  "Q0`"
  oregbr1/1 -> Shifting Logic6/8(dlsb), Shifting Logic7/1(lsb)
  oregbr0/1 -> Shifting Logic7/8(dlsb)
  oregbl0/1 -> Shifting Logic2/7(drsb), Shifting Logic/6(rsb)
  oregbl1/1 -> Shifting Logic/7(drsb)

== system Block Diagram/ALU/all_equal_a ==
  in0 : Inport
  in1 : Inport  Port=2
  in2 : Inport  Port=3
  AND : Logic  IconShape=distinctive  AllPortsSameDT=off  OutDataTypeStr=boolean
  NOT1 : Logic  Operator=NOT  IconShape=distinctive  AllPortsSameDT=off  OutDataTypeStr=boolean
  NOT2 : Logic  Operator=NOT  IconShape=distinctive  AllPortsSameDT=off  OutDataTypeStr=boolean
  XOR : Logic  Operator=XOR  IconShape=distinctive  AllPortsSameDT=off  OutDataTypeStr=boolean
  XOR1 : Logic  Operator=XOR  IconShape=distinctive  AllPortsSameDT=off  OutDataTypeStr=boolean
  all_equal : Outport
  wires:
  AND/1 -> all_equal/1
  in2/1 -> XOR1/2
  in1/1 -> XOR1/1, XOR/2
  in0/1 -> XOR/1
  XOR1/1 -> NOT1/1
  XOR/1 -> NOT2/1
  NOT2/1 -> AND/1
  NOT1/1 -> AND/2

== system Block Diagram/ALU/all_equal_q ==
  in0 : Inport
  in1 : Inport  Port=2
  in2 : Inport  Port=3
  AND : Logic  IconShape=distinctive  AllPortsSameDT=off  OutDataTypeStr=boolean
  NOT1 : Logic  Operator=NOT  IconShape=distinctive  AllPortsSameDT=off  OutDataTypeStr=boolean
  NOT2 : Logic  Operator=NOT  IconShape=distinctive  AllPortsSameDT=off  OutDataTypeStr=boolean
  XOR : Logic  Operator=XOR  IconShape=distinctive  AllPortsSameDT=off  OutDataTypeStr=boolean
  XOR1 : Logic  Operator=XOR  IconShape=distinctive  AllPortsSameDT=off  OutDataTypeStr=boolean
  all_equal : Outport
  wires:
  AND/1 -> all_equal/1
  in2/1 -> XOR1/2
  in1/1 -> XOR1/1, XOR/2
  in0/1 -> XOR/1
  XOR1/1 -> NOT1/1
  XOR/1 -> NOT2/1
  NOT2/1 -> AND/1
  NOT1/1 -> AND/2

== system Block Diagram/ALU/cnt1 ==
  clk : Inport
  rst : Inport  Port=2
  3-bit counter : Subsystem
  AND : Logic  Inputs=3  IconShape=distinctive  AllPortsSameDT=off  OutDataTypeStr=boolean
  AND1 : Logic  Inputs=3  IconShape=distinctive  AllPortsSameDT=off  OutDataTypeStr=boolean
  NOT : Logic  Operator=NOT  IconShape=distinctive  AllPortsSameDT=off  OutDataTypeStr=boolean
  NOT1 : Logic  Operator=NOT  IconShape=distinctive  AllPortsSameDT=off  OutDataTypeStr=boolean
  cnt4 : Outport
  cnt7 : Outport  Port=2
  wires:
  clk/1 -> 3-bit counter/1(clk)
  rst/1 -> 3-bit counter/2(rst)
  3-bit counter/3(b2) -> AND1/3, AND/3
  AND/1 -> cnt7/1
  NOT/1 -> AND1/1
  NOT1/1 -> AND1/2
  AND1/1 -> cnt4/1
  3-bit counter/1(b0) -> AND/1, NOT/1
  3-bit counter/2(b1) -> AND/2, NOT1/1

== system Block Diagram/ALU/cnt2 ==
  count_down : Inport
  count_up : Inport  Port=2
  rst : Inport  Port=3
  clk : Inport  Port=4
  3-bit counter : Subsystem
  3-bit counter1 : Subsystem
  AND : Logic  IconShape=distinctive  AllPortsSameDT=off  OutDataTypeStr=boolean
  AND1 : Logic  IconShape=distinctive  AllPortsSameDT=off  OutDataTypeStr=boolean
  NOR : Logic  Operator=NOR  Inputs=3  IconShape=distinctive  AllPortsSameDT=off  OutDataTypeStr=boolean
  XOR : Logic  Operator=XOR  IconShape=distinctive  AllPortsSameDT=off  OutDataTypeStr=boolean
  XOR1 : Logic  Operator=XOR  IconShape=distinctive  AllPortsSameDT=off  OutDataTypeStr=boolean
  XOR2 : Logic  Operator=XOR  IconShape=distinctive  AllPortsSameDT=off  OutDataTypeStr=boolean
  cnt0 : Outport
  wires:
  rst/1 -> 3-bit counter1/1(rst), 3-bit counter/2(rst)
  count_up/1 -> AND/1
  clk/1 -> AND1/1, AND/2
  AND1/1 -> 3-bit counter1/2(clk)
  count_down/1 -> AND1/2
  AND/1 -> 3-bit counter/1(clk)
  3-bit counter/1(b0) -> XOR2/1
  3-bit counter1/1(b0) -> XOR2/2
  3-bit counter1/2(b1) -> XOR1/2
  3-bit counter/2(b1) -> XOR1/1
  3-bit counter1/3(b2) -> XOR/2
  3-bit counter/3(b2) -> XOR/1
  XOR2/1 -> NOR/1
  XOR/1 -> NOR/3
  XOR1/1 -> NOR/2
  NOR/1 -> cnt0/1
